simulink model "CicloAperto"  (R2023b)
settings: Solver=VariableStepAuto  StartTime=0.0  StopTime=100.0  MaxStep=0.1  RelTol=1e-6
settings Model: Creator=adamo  LastModifiedBy=franc

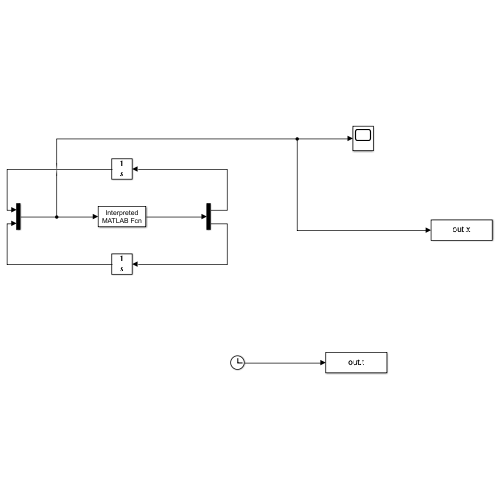
[thumbnail: Simulink's stored preview of the top-level diagram]
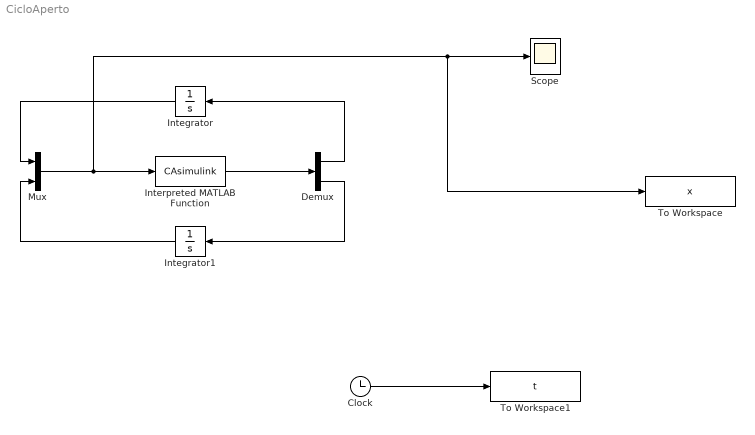
== system CicloAperto ==
  Clock : Clock
  Demux : Demux  Outputs=2
  Integrator : Integrator  InitialCondition=0.5
  Integrator1 : Integrator
  Interpreted MATLAB Function : MATLABFcn  MATLABFcn=CAsimulink  OutputDimensions=2
  Mux : Mux  Inputs=2
  Scope : Scope
  To Workspace : ToWorkspace  VariableName=x  SampleTime=-1
  To Workspace1 : ToWorkspace  VariableName=t  SampleTime=-1
  wires:
  Interpreted MATLAB Function/1 -> Demux/1
  Demux/1 -> Integrator/1
  Integrator/1 -> Mux/1
  Integrator1/1 -> Mux/2
  Demux/2 -> Integrator1/1
  Mux/1 -> To Workspace/1, Scope/1, Interpreted MATLAB Function/1
  Clock/1 -> To Workspace1/1
